simulink model "buck_adc_noise_duty_jitter_logic"  (R2024b)
settings: Solver=ode4  StartTime=0.0  StopTime=0.020  FixedStep=5e-7  RelTol=1e-3
settings Model: Creator=ww  LastModifiedBy=ww

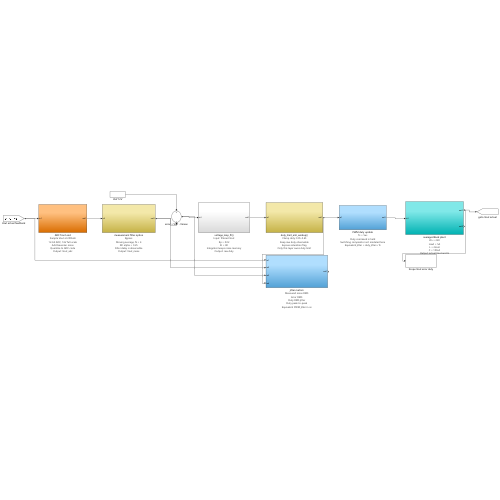
[thumbnail: Simulink's stored preview of the top-level diagram]
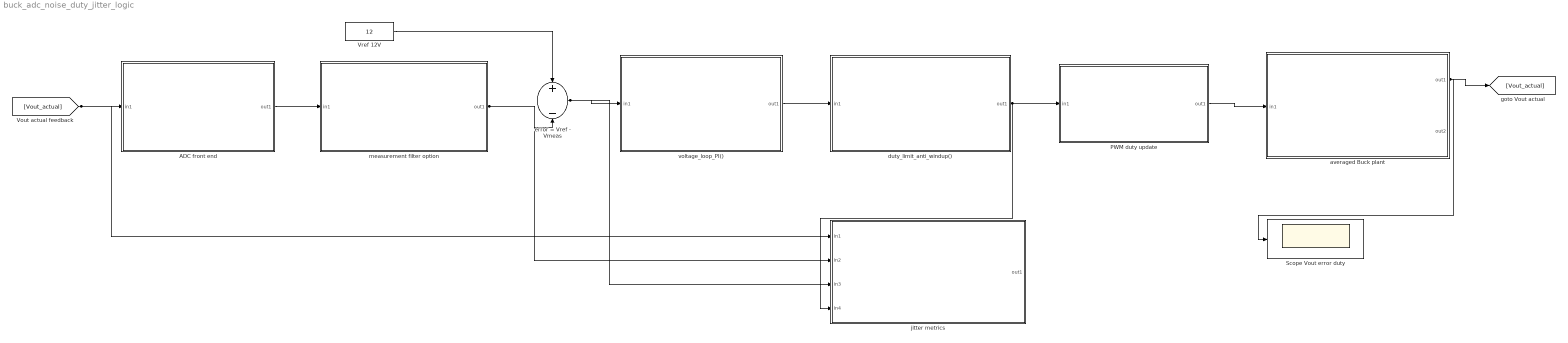
== system buck_adc_noise_duty_jitter_logic ==
  ADC front end : Subsystem
      settings: AttributesFormatString=|
      | Sample Vout at 200kHz
      | 12-bit ADC, 16V full-scale
      | Add Gaussian noise
      | Quantize to ADC code
      | Output: Vout_adc
  PWM duty update : Subsystem
      settings: AttributesFormatString=|
      | Ts = 5us
      | Duty command is held
      | Switching comparator not modeled here
      | Equivalent jitter = duty jitter x Ts
  Scope Vout error duty : Scope
  Vref 12V : Constant  Value=12
  averaged Buck plant : Subsystem
      settings: AttributesFormatString=|
      | Vin = 24V
      | Load = 5A
      | L = 22uH
      | C = 100uF
      | Output: actual Vout and IL
  duty_limit_anti_windup() : Subsystem
      settings: AttributesFormatString=|
      | Clamp duty: 0.05..0.65
      | Keep raw duty observable
      | Expose saturation flag
      | Only this layer owns duty limit
  error = Vref - Vmeas : Sum  Inputs=+-
  jitter metrics : Subsystem
      settings: AttributesFormatString=|
      | Measured noise RMS
      | Error RMS
      | Duty RMS jitter
      | Duty peak-to-peak
      | Equivalent PWM jitter in ns
  measurement filter option : Subsystem
      settings: AttributesFormatString=|
      | Bypass
      | Moving average, N = 4
      | IIR: alpha = 0.25
      | Filter delay is observable
      | Output: Vout_meas
  voltage_loop_PI() : Subsystem
      settings: AttributesFormatString=|
      | Input: filtered Vout
      | Kp = 0.02
      | Ki = 80
      | Integrator keeps noise memory
      | Output: raw duty
  wires:
  [Vout_actual] -> ADC front end/1(in1), jitter metrics/1(in1)
  ADC front end/1(out1) -> measurement filter option/1(in1)
  measurement filter option/1(out1) -> error = Vref - Vmeas/2, jitter metrics/2(in2)
  Vref 12V/1 -> error = Vref - Vmeas/1
  error = Vref - Vmeas/1 -> voltage_loop_PI()/1(in1), jitter metrics/3(in3)
  voltage_loop_PI()/1(out1) -> duty_limit_anti_windup()/1(in1)
  duty_limit_anti_windup()/1(out1) -> PWM duty update/1(in1), jitter metrics/4(in4)
  PWM duty update/1(out1) -> averaged Buck plant/1(in1)
  averaged Buck plant/1(out1) -> [Vout_actual], Scope Vout error duty/1

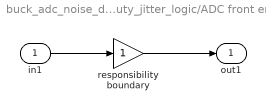
== system buck_adc_noise_duty_jitter_logic/ADC front end ==
  in1 : Inport
  responsibility boundary : Gain  Description=|
      | Sample Vout at 200kHz
      | 12-bit ADC, 16V full-scale
      | Add Gaussian noise
      | Quantize to ADC code
      | Output: Vout_adc
  out1 : Outport
  wires:
  in1/1 -> responsibility boundary/1
  responsibility boundary/1 -> out1/1

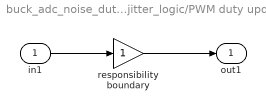
== system buck_adc_noise_duty_jitter_logic/PWM duty update ==
  in1 : Inport
  responsibility boundary : Gain  Description=|
      | Ts = 5us
      | Duty command is held
      | Switching comparator not modeled here
      | Equivalent jitter = duty jitter x Ts
  out1 : Outport
  wires:
  responsibility boundary/1 -> out1/1
  in1/1 -> responsibility boundary/1

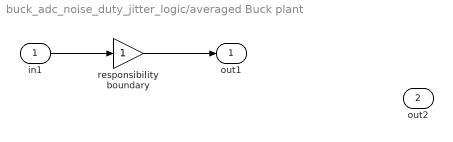
== system buck_adc_noise_duty_jitter_logic/averaged Buck plant ==
  in1 : Inport
  responsibility boundary : Gain  Description=|
      | Vin = 24V
      | Load = 5A
      | L = 22uH
      | C = 100uF
      | Output: actual Vout and IL
  out1 : Outport
  out2 : Outport  Port=2
  wires:
  in1/1 -> responsibility boundary/1
  responsibility boundary/1 -> out1/1

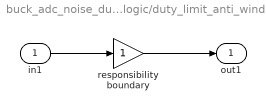
== system buck_adc_noise_duty_jitter_logic/duty_limit_anti_windup() ==
  in1 : Inport
  responsibility boundary : Gain  Description=|
      | Clamp duty: 0.05..0.65
      | Keep raw duty observable
      | Expose saturation flag
      | Only this layer owns duty limit
  out1 : Outport
  wires:
  responsibility boundary/1 -> out1/1
  in1/1 -> responsibility boundary/1

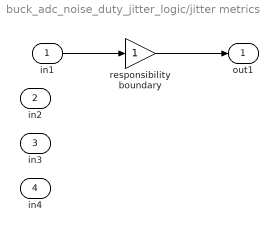
== system buck_adc_noise_duty_jitter_logic/jitter metrics ==
  in1 : Inport
  in2 : Inport  Port=2
  in3 : Inport  Port=3
  in4 : Inport  Port=4
  responsibility boundary : Gain  Description=|
      | Measured noise RMS
      | Error RMS
      | Duty RMS jitter
      | Duty peak-to-peak
      | Equivalent PWM jitter in ns
  out1 : Outport
  wires:
  responsibility boundary/1 -> out1/1
  in1/1 -> responsibility boundary/1

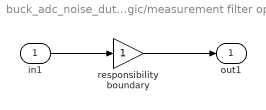
== system buck_adc_noise_duty_jitter_logic/measurement filter option ==
  in1 : Inport
  responsibility boundary : Gain  Description=|
      | Bypass
      | Moving average, N = 4
      | IIR: alpha = 0.25
      | Filter delay is observable
      | Output: Vout_meas
  out1 : Outport
  wires:
  responsibility boundary/1 -> out1/1
  in1/1 -> responsibility boundary/1

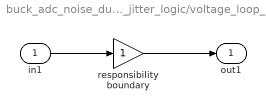
== system buck_adc_noise_duty_jitter_logic/voltage_loop_PI() ==
  in1 : Inport
  responsibility boundary : Gain  Description=|
      | Input: filtered Vout
      | Kp = 0.02
      | Ki = 80
      | Integrator keeps noise memory
      | Output: raw duty
  out1 : Outport
  wires:
  in1/1 -> responsibility boundary/1
  responsibility boundary/1 -> out1/1
